simulink model "PortSelection"  (R2020a)
settings: Solver=FixedStepDiscrete  StartTime=0.0  StopTime=SIM_TIME  FixedStep=10e-6  RelTol=1e-3
PreLoadFcn:
  | SIM_TIME = 15
libraries: powerlib x1
settings Model: Creator=debma  LastModifiedBy=debma

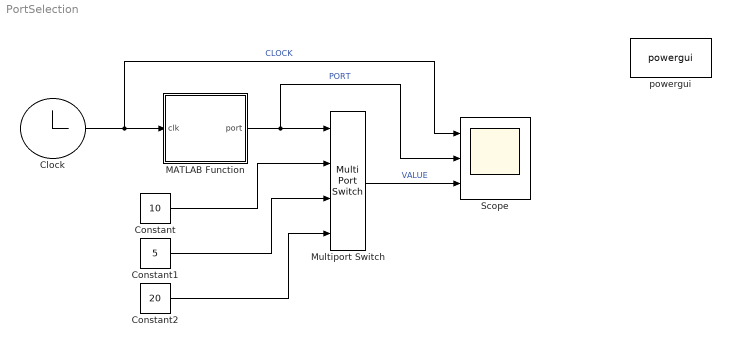
== system PortSelection ==
  Clock : Clock
  Constant : Constant  Value=10
  Constant1 : Constant  Value=5
  Constant2 : Constant  Value=20
  MATLAB Function : MATLAB Function  TreatAsAtomicUnit=on
  Multiport Switch : MultiPortSwitch
  Scope : Scope  NumInputPorts=3
  powergui : powerlib/powergui  Priority=1  SimulationMode=Discrete  SampleTime=10e-6  frequency=60  Iterations=50  frequencyindice=60  Pbase=100e6  ErrMax=1e-4  UnitsV=kV  UnitsW=MW  buscounter=0  FunctionMessages=off  echomessages=off  EnableUseOfTLC=off  CurrentSourceSwitches=off  DisableSnubberDevices=off  DisableRonSwitches=off  DisableVfSwitches=off  DisplayEquations=off  AutomaticDiscreteSolvers=off  SolverType=Tustin/Backward Euler (TBE)  Interpol=off  ExternalGateDelay=off  methode=off  Ts=100  x0status=blocks  SPID=on  SwTol=0  HookPort=off  NonlinearTolerance=1e-4  nMaxIteration=100  ContinueOnMaxIteration=off  RestoreLinks=warning  ResistiveCurrentMeasurement=off  Frange=[0:2:500]  Ylog=off  Xlog=on  ShowGrid=off  save=off  variable=ZData  structure=0  ZoomFFT=off  StartTime=0.0  cycles=1  DisplayStyle=1  fundamental=60  FreqAxis=off  MaxFrequency=1000  frequencyindicesteady=1  RmsSteady=1  display=off
  wires:
  Clock/1 -> Scope/1, MATLAB Function/1(clk)  "CLOCK"
  MATLAB Function/1(port) -> Scope/2, Multiport Switch/1  "PORT"
  Multiport Switch/1 -> Scope/3  "VALUE"
  Constant/1 -> Multiport Switch/2
  Constant1/1 -> Multiport Switch/3
  Constant2/1 -> Multiport Switch/4

== matlab function PortSelection/MATLAB Function ==
  data: clk input; port output
%% A Function to select different port of Multi-Port Switch
function port = PortSelection(clk)
    % Given the Simulation-Clock and Multi-Port Switch, with 3-Cases
    % this function divides the total simulation time into 3-interval
    % and based on it, activates the multi-port switch
    % uses the variable SIM_TIME
    % defined in Model Callbacks
    
    if clk <= 5
        port = 1;
    elseif clk > 5 && clk < 10
        port = 2;
    else
        port = 3;
    end
